simulink model "discrete_time_ground_vehicle_simulation"  (R2024a)
settings: Solver=VariableStepAuto  StartTime=0.0  StopTime=10.0  RelTol=1e-3
model workspace (MAT data in the model file):
  x0 = Simulink.Parameter
  x0.Value = [0; 0; 0]
  x0.Complexity = 'real'
  x0.Dimensions = [3 1]
  x0.DataType = 'auto'
libraries: SignalEditorBlockLib x1
settings Model: Creator=venkat  LastModifiedBy=venkat
settings DataIOCC: InitialState=[1,1,0]  LoadInitialState=on

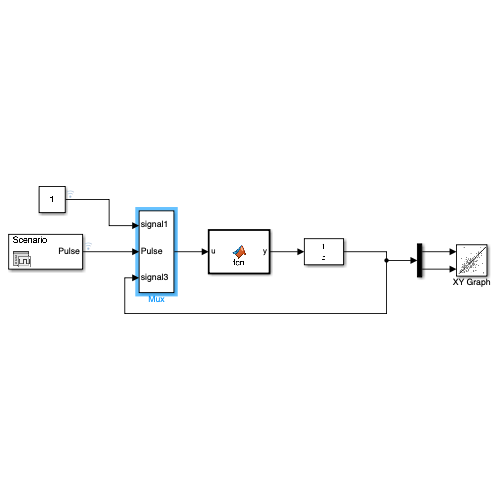
[thumbnail: Simulink's stored preview of the top-level diagram]
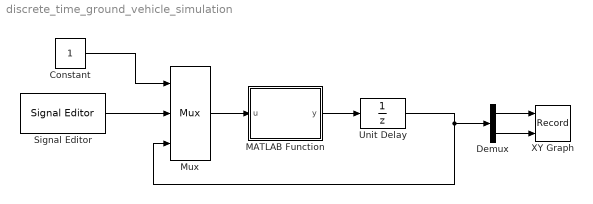
== system discrete_time_ground_vehicle_simulation ==
  Constant : Constant
  Demux : Demux  Outputs=2
  MATLAB Function : MATLAB Function  TreatAsAtomicUnit=on
  Mux : Mux  Inputs=3
      settings: DisplayOption=signals
  Signal Editor : SignalEditorBlockLib/Signal Editor  FileName=pulse_signal.mat  ActiveScenario=Scenario  ActiveSignal=Pulse  IsBus=off  OutputBusObjectStr=Bus: BusObject  SampleTime=0  Interpolate=off  ZeroCross=off  OutputAfterFinalValue=Setting to zero  Unit=inherit  PreserveSignalName=on  ApplySigPropsToAllScenarios=on  ApplySigPropsToAllSignals=off
  Unit Delay : UnitDelay  InitialCondition=x0  SampleTime=0.1  HasFrameUpgradeWarning=on
  XY Graph : Record  FileSettingsInternal="{\"entries\":[{\"content\":{\"excelSettings\":{\"content\":{},\"type\":\"Streamout.ExcelSettings\"}},\"type\":\"Streamout.FileSettingStorage\",\"uuid\":\"\"}],\"packageUris\":[\"http:\\/\\/schema.mathworks.com\\/mf0\\/streamout_blocks\\/R2020a\"],\"version\":\"1.0\"}"  Layout=[1 1]  SignalsInternal="{\"entries\":[{\"content\":{\"signals\":[{\"content\":{\"blockPath\":[],\"dimensions\":[2,1],\"domain\":\"\",\"hasChildren\":true,\"lineColor\":\"#d95319\",\"lineWidth\":2,\"port\":1,\"sid\":[\"\"],\"signalID\":1},\"type\":\"RecordBlkView.Signal\",\"uuid\":\"\"},{\"content\":{\"blockPath\":[],\"channel\":[1,1],\"dimensions\":[2,1],\"domain\":\"\",\"lineColor\":\"#edb120\",\"lineWidth\":2,\"parentID\":1,\"plots\":[ 1 ],\"port\":1,\"sid\":[\"\"],\"signalID\":2},\"type\":\"RecordBlkView.Signal\",\"uuid\":\"\"},{\"content\":{\"blockPath\":[],\"dimensions\":[1,1],\"domain\":\"\",\"lineColor\":\"#7e2f8e\",\"lineWidth\":2,\"port\":2,\"sid\":[\"\"],\"signalID\":3,\"signalName\":\"Demux:2\"},\"type\":\"RecordBlkView.Signal\",\"uuid\":\"\"},{\"content\":{\"blockPath\":[],\"channel\":[2,1],\"dimensions\":[2,1],\"domain\":\"\",\"lineColor\":\"#a2142f\",\"lineWidth\":2,\"parentID\":1,\"plots\":[ 1 ],\"port\":1,\"sid\":[\"\"],\"signalID\":4},\"type\":\"RecordBlkView.Signal\",\"uuid\":\"\"}]},\"type\":\"RecordBlkView.InputSignals\",\"uuid\":\"\"}],\"packageUris\":[\"http:\\/\\/schema.mathworks.com\\/mf0\\/streamout_blocks\\/R2020a\"],\"version\":\"1.0\"}"  VisualizationBindings="{\"xyplotplugin\":{\"info\":[{\"series\":[{\"bindingParametersList\":[{\"parameter\":\"X-Axis\",\"signalID\":2,\"signalName\":\"Demux:1(1,1)\"},{\"parameter\":\"Y-Axis\",\"signalID\":4,\"signalName\":\"Demux:1(2,1)\"},{\"parameter\":\"X-Axis\",\"signalID\":2,\"signalName\":\"Demux:1(1,1)\"},{\"parameter\":\"X-Axis\",\"signalID\":2,\"signalName\":\"Demux:1(1,1)\"},{\"parameter\":\"Y-Axis\",\"signalID\":4,\"signalName\":\"Demux:1(2,1)\"}],\"seriesID\":0},{\"bindingParametersList\":[{\"parameter\":\"X-Axis\",\"signalID\":4,\"signalName\":\"Demux:1(2,1)\"}],\"seriesID\":1}],\"subplotID\":1}]}}"  CompatibilityTag=XY
  wires:
  MATLAB Function/1(y) -> Unit Delay/1
  Constant/1 -> Mux/1
  Unit Delay/1 -> Mux/3, Demux/1
  Signal Editor/1 -> Mux/2
  Mux/1 -> MATLAB Function/1(u)
  Demux/1 -> XY Graph/1
  Demux/2 -> XY Graph/2

== matlab function discrete_time_ground_vehicle_simulation/MATLAB Function ==
  data: u input; y output
function y = fcn(u)

% parse u variable and assign them to state vars and local vars.
v1 = u(1);
v2 = u(2);
x1 = u(3);
x2 = u(4);
x3 = u(5);

% parameters
d = 0.01;
c = 0.1;

%definition of g
x1next = x1 + d*sin(x3)*v1;
x2next = x2 + d*cos(x3)*v1;
x3next = x3 + c*v2;

disp([x1 x2 x3])

y = [x1next;x2next;x3next];
